simulink model "ADCSWorkshop2026_6DOFSim"  (R2026a)
settings: Solver=FixedStepAuto  StopTime=36000  FixedStep=1
values from neighbouring files (symbols this model uses):
  attitudeState0 = [q0' w0']'    [SimInitializer.m]
  inertia = diag([0.05 0.05 0.01])    [SimInitializer.m]
  muEarth = 3.986004418e5    (= 398600.4418)    [SimInitializer.m]
  orbitState0 = [r0; v0]    [SimInitializer.m]
undefined symbols (not defined in the file or in its folder): IAU
libraries: aerolibtransform2 x1
settings Model: Creator=justi  LastModifiedBy=Celeste

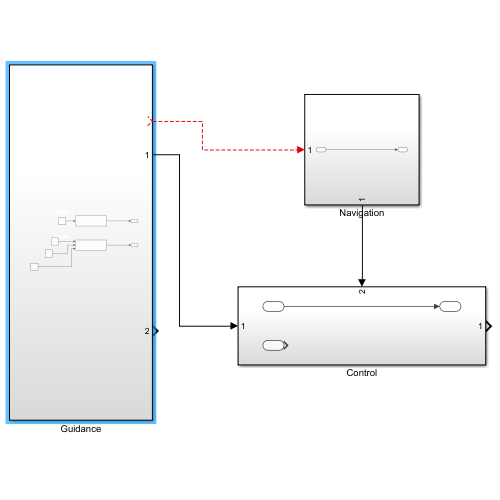
[thumbnail: Simulink's stored preview of the top-level diagram]
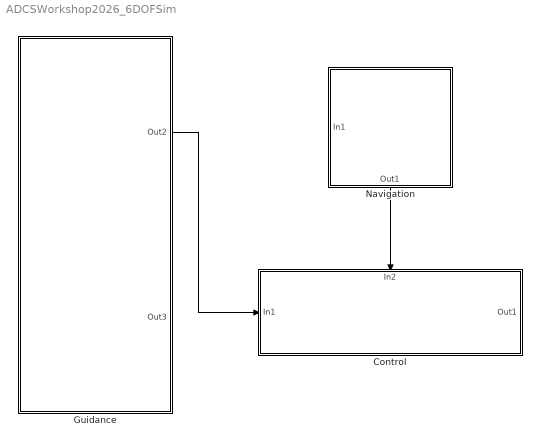
== system ADCSWorkshop2026_6DOFSim ==
  Control : Subsystem
      settings: PortSchema="{\"entries\":[{\"content\":{\"sides\":[{\"content\":{\"connectorIds\":[\"In1\"]},\"type\":\"ConnectorPlacement.EquallySpacedRectSide\",\"uuid\":\"45a25749-5a66-47ef-a74b-952d4e64ae75\"},{\"content\":{\"connectorIds\":[\"Out1\"],\"side\":\"RIGHT\"},\"type\":\"ConnectorPlacement.EquallySpacedRectSide\",\"uuid\":\"248e7eff-17cc-4f29-a0d8-747ed88f9ef8\"},{\"content\":{\"connectorIds\":[\"In2\"],\"side\":\"TOP\"},\"type\":\"ConnectorPlacement.EquallySpacedRectSide\",\"uuid\":\"9f62952b-b28e-4367-83ff-4c76f4ba2b72\"}]},\"type\":\"ConnectorPlacement.EquallySpacedConnector\",\"uuid\":\"2205c168-d106-415a-b3b2-56bec6f8c213\"}],\"packageUris\":[\"http://schema.mathworks.com/mf0/Connector/R2020b\"],\"version\":\"1.0\"}"
  Guidance : Subsystem
  Navigation : Subsystem
      settings: PortSchema="{\"entries\":[{\"content\":{\"sides\":[{\"content\":{\"connectorIds\":[\"In1\"]},\"type\":\"ConnectorPlacement.EquallySpacedRectSide\",\"uuid\":\"22603658-6c40-48e3-8114-7b85dabb1b7c\"},{\"content\":{\"side\":\"RIGHT\"},\"type\":\"ConnectorPlacement.EquallySpacedRectSide\",\"uuid\":\"0066126e-5306-4c26-b788-27481a70a8d4\"},{\"content\":{\"side\":\"TOP\"},\"type\":\"ConnectorPlacement.EquallySpacedRectSide\",\"uuid\":\"f42b0298-09c7-435c-abc1-4550c46c52f1\"},{\"content\":{\"connectorIds\":[\"Out1\"],\"side\":\"BOTTOM\"},\"type\":\"ConnectorPlacement.EquallySpacedRectSide\",\"uuid\":\"255cde04-3dec-4ac2-8b3c-05db596d1a27\"}]},\"type\":\"ConnectorPlacement.EquallySpacedConnector\",\"uuid\":\"39e9370b-3b87-44ed-bba4-5c794c2b66b9\"}],\"packageUris\":[\"http://schema.mathworks.com/mf0/Connector/R2020b\"],\"version\":\"1.0\"}"
  wires:
  Navigation/1(Out1) -> Control/2(In2)
  Guidance/1(Out2) -> Control/1(In1)
  ? -> Navigation/1(In1)

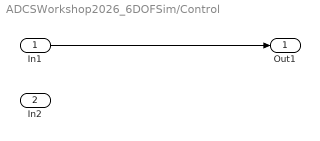
== system ADCSWorkshop2026_6DOFSim/Control ==
  In1 : Inport
  In2 : Inport  Port=2
  Out1 : Outport
  wires:
  In1/1 -> Out1/1

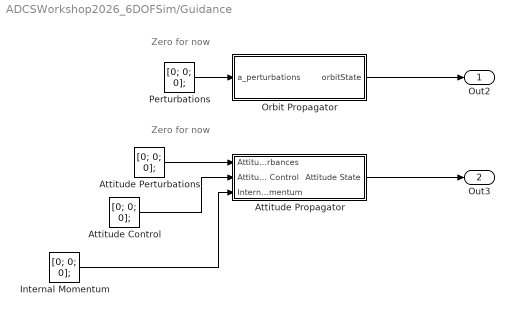
== system ADCSWorkshop2026_6DOFSim/Guidance ==
  note: Zero for now
  note: Zero for now
  Attitude Control : Constant  Value=[0; 0; 0];
  Attitude Perturbations : Constant  Value=[0; 0; 0];
  Attitude Propagator : Subsystem
  Internal Momentum : Constant  Value=[0; 0; 0];
  Orbit Propagator : Subsystem
  Perturbations : Constant  Value=[0; 0; 0];
  Out2 : Outport
  Out3 : Outport  Port=2
  wires:
  Orbit Propagator/1(orbitState) -> Out2/1
  Perturbations/1 -> Orbit Propagator/1(a_perturbations)
  Attitude Perturbations/1 -> Attitude Propagator/1(Attitude Disturbances)
  Attitude Propagator/1(Attitude State) -> Out3/1
  Attitude Control/1 -> Attitude Propagator/2(Attitude Control)
  Internal Momentum/1 -> Attitude Propagator/3(Internal Momentum)

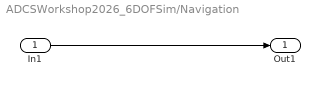
== system ADCSWorkshop2026_6DOFSim/Navigation ==
  In1 : Inport
  Out1 : Outport
  wires:
  In1/1 -> Out1/1

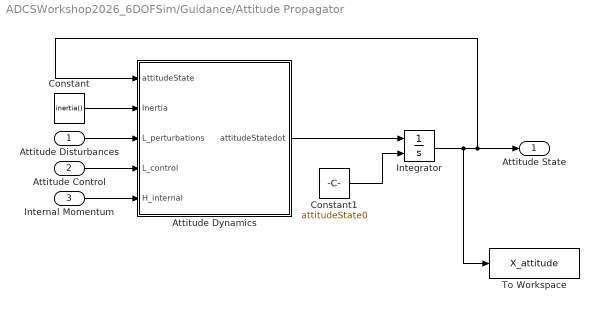
== system ADCSWorkshop2026_6DOFSim/Guidance/Attitude Propagator ==
  Attitude Disturbances : Inport
  Attitude Control : Inport  Port=2
  Internal Momentum : Inport  Port=3
  Attitude Dynamics : MATLAB Function  TreatAsAtomicUnit=on
  Constant : Constant  Value=inertia()
  Constant1 : Constant  Value=attitudeState0  VectorParams1D=off
  Integrator : Integrator  InitialConditionSource=external
  To Workspace : ToWorkspace  VariableName=X_attitude  SaveFormat=Timeseries  SampleTime=-1
  Attitude State : Outport
  wires:
  Attitude Dynamics/1(attitudeStatedot) -> Integrator/1
  Attitude Disturbances/1 -> Attitude Dynamics/3(L_perturbations)
  Constant/1 -> Attitude Dynamics/2(Inertia)
  Constant1/1 -> Integrator/2
  Integrator/1 -> To Workspace/1, Attitude Dynamics/1(attitudeState), Attitude State/1
  Attitude Control/1 -> Attitude Dynamics/4(L_control)
  Internal Momentum/1 -> Attitude Dynamics/5(H_internal)

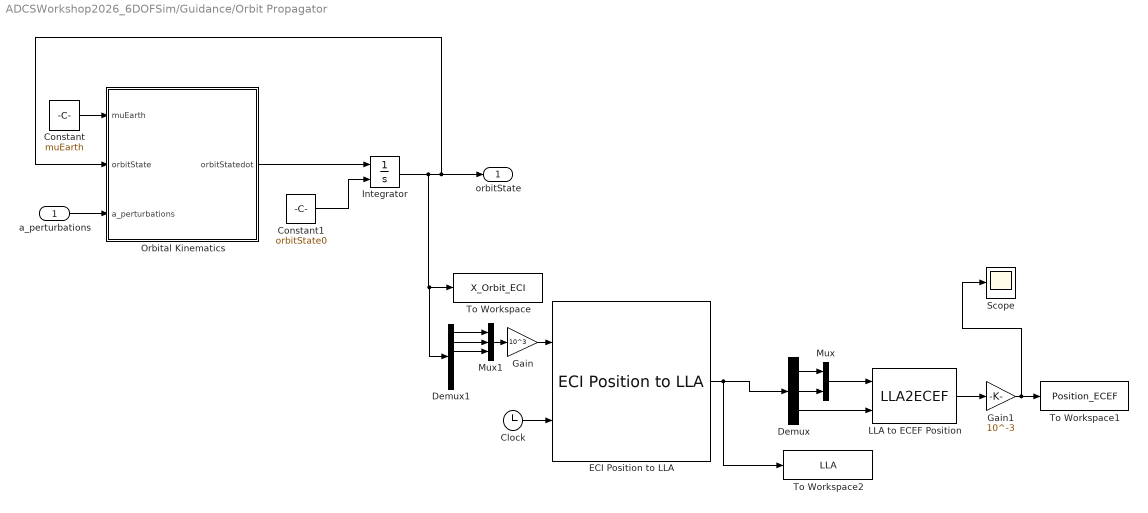
== system ADCSWorkshop2026_6DOFSim/Guidance/Orbit Propagator ==
  a_perturbations : Inport
  Clock : Clock
  Constant : Constant  Value=muEarth
  Constant1 : Constant  Value=orbitState0  VectorParams1D=off
  Demux : Demux  Outputs=3
  Demux1 : Demux  Outputs=6
  ECI Position to LLA : aerolibtransform2/ECI Position to LLA  red=IAU-2000/2006  year=2024  month=March  day=10  hour=7  min=0  sec=0  deltaT=Sec  errorflag=Error  extraparamflag=off  eunits=Metric (MKS)  earthmodel=WGS84  flat=1/298.257223563  eqradius=6378137
      settings: AttributesFormatString=%<red>
  Gain : Gain  Gain=10^3
  Gain1 : Gain  Gain=10^-3
  Integrator : Integrator  InitialConditionSource=external
  LLA to ECEF Position : LLA2ECEF
  Mux : Mux  Inputs=2
  Mux1 : Mux  Inputs=3
  Orbital Kinematics : MATLAB Function  TreatAsAtomicUnit=on
  Scope : Scope
      settings: ActiveDisplayYMinimum=-1  ActiveDisplayYMaximum=1
  To Workspace : ToWorkspace  VariableName=X_Orbit_ECI  SaveFormat=Timeseries  SampleTime=-1
  To Workspace1 : ToWorkspace  VariableName=Position_ECEF  SaveFormat=Timeseries  SampleTime=-1
  To Workspace2 : ToWorkspace  VariableName=LLA  SaveFormat=Timeseries  SampleTime=-1
  orbitState : Outport
  wires:
  Orbital Kinematics/1(orbitStatedot) -> Integrator/1
  a_perturbations/1 -> Orbital Kinematics/3(a_perturbations)
  Constant/1 -> Orbital Kinematics/1(muEarth)
  Constant1/1 -> Integrator/2
  ECI Position to LLA/1 -> To Workspace2/1, Demux/1
  Demux/1 -> Mux/1
  Demux/2 -> Mux/2
  Mux/1 -> LLA to ECEF Position/1
  Demux/3 -> LLA to ECEF Position/2
  LLA to ECEF Position/1 -> Gain1/1
  Demux1/2 -> Mux1/2
  Demux1/1 -> Mux1/1
  Demux1/3 -> Mux1/3
  Clock/1 -> ECI Position to LLA/2
  Integrator/1 -> Demux1/1, To Workspace/1, Orbital Kinematics/2(orbitState), orbitState/1
  Mux1/1 -> Gain/1
  Gain/1 -> ECI Position to LLA/1
  Gain1/1 -> Scope/1, To Workspace1/1

== matlab function ADCSWorkshop2026_6DOFSim/Guidance/Attitude Propagator/Attitude Dynamics ==
  data: attitudeState input; Inertia input; attitudeStatedot output; L_perturbations input; L_control input; H_internal input
function attitudeStatedot = AttitudeDynamics(attitudeState, Inertia, L_perturbations, L_control, H_internal)
    % Extract state values
    % q : quaternion [] (4,1)
    % w : angular velocity [rad/s] (3,1)
    q = attitudeState(1:4);
    w = attitudeState(5:7);

    % Quaternion dynamics (temporarily disabled)
    q_dot = zeros(4,1);

    % Rotational dynamics
    w_dot = Inertia \ (L_perturbations + L_control ...
        - cross(w, Inertia*w + H_internal));

    attitudeStatedot = [q_dot; w_dot];
end

== matlab function ADCSWorkshop2026_6DOFSim/Guidance/Orbit Propagator/Orbital Kinematics ==
  data: muEarth input; orbitState input; orbitStatedot output; a_perturbations input
function orbitStatedot  = OrbitKinematics(muEarth, orbitState, a_perturbations)
    % Extract state orbitState values
    % r : position [km]
    % v : velocity [km/s]
    r_eci = orbitState(1:3);
    r_mag = sqrt(orbitState(1)^2 + orbitState(2)^2 + orbitState(3)^2);
    v_eci = orbitState(4:6);
    
    % Two-body Equations of Motion
    rdot = v_eci;
    vdot = -muEarth/r_mag^3 * r_eci + a_perturbations;
    
    orbitStatedot = [rdot;
                     vdot];
end
